simulink model "WEEK1_QN8"  (R2020b)
settings: Solver=VariableStepAuto  StartTime=0.0  StopTime=10.0  RelTol=1e-3
settings Model: Creator=dell  LastModifiedBy=dell

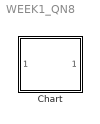
== system WEEK1_QN8 ==
  Chart : Stateflow chart  TreatAsAtomicUnit=on

== stateflow chart WEEK1_QN8/Chart ==
  state Floor5
    entry:
    mode=1;
    during:
    current_floor=5;
    presentFloor(current_floor);
    exit:
    mode=0;
  state Floor4
    entry:
    mode=1;
    during:
    current_floor=4;
    presentFloor(current_floor);
    exit:
    mode=0;
  state Floor3
    entry:
    mode=1;
    during:
    current_floor=3;
    presentFloor(current_floor);
    exit:
    mode=0;
  state Floor2
    entry:
    mode=1;
    during:
    current_floor=2;
    presentFloor(current_floor);
    exit:
    mode=0;
  state Floor1
    entry:
    mode=1;
    during:
    current_floor=1;
    presentFloor(current_floor);
    exit:
    mode=0;
  state Floor0
    entry:
    mode=1;
    during:
    current_floor=0;
    presentFloor(current_floor);
    exit:
    mode=0;
  Floor5 -> Floor4 : descend
  Floor4 -> Floor5 [order 1] : ascend
  Floor4 -> Floor3 [order 2] : descend
  Floor3 -> Floor4 [order 2] : ascend
  Floor3 -> Floor2 [order 1] : descend
  Floor2 -> Floor3 [order 1] : ascend
  Floor2 -> Floor1 [order 2] : descend
  Floor1 -> Floor2 [order 2] : ascend
  Floor1 -> Floor0 [order 1] : descend
  Floor0 -> Floor1 : ascend
  (default) -> Floor0
  data: presentFloor input; mode output; current_floor local
  events: ascend local RISING_EDGE_EVENT; descend local RISING_EDGE_EVENT
